simulink model "linealidad"  (R2020b)
settings: Solver=VariableStepAuto  StartTime=0.0  StopTime=5  RelTol=1e-3
settings Model: Creator=carma  LastModifiedBy=carma

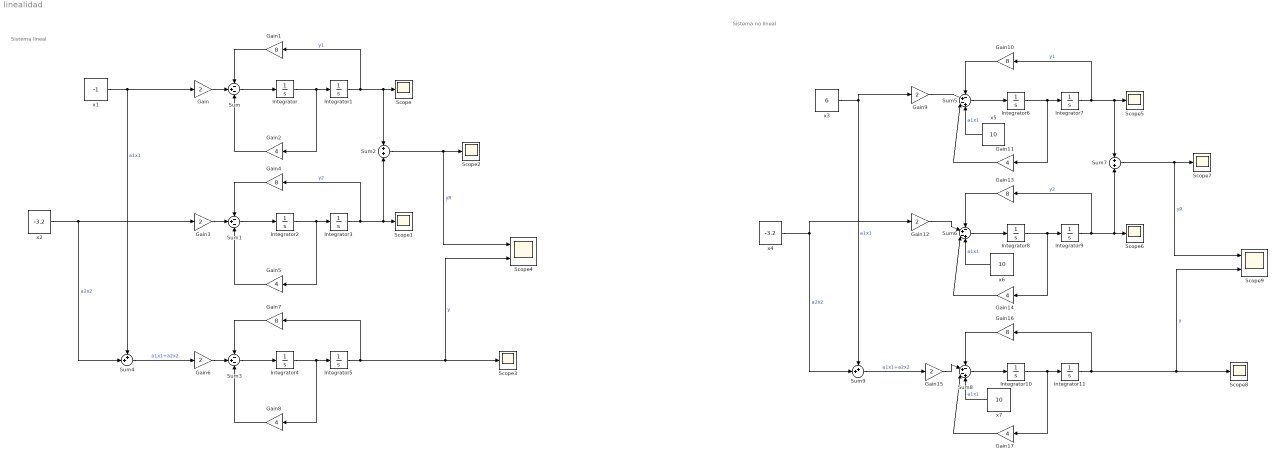
== system linealidad ==
  note: Sistema no lineal
  note: Sistema lineal
  Gain{,3,6,9,12,15} (6 alike) : Gain  Gain=2
  Gain{1,4,7,10,13,16} (6 alike) : Gain  Gain=8
  Gain{2,5,8,11,14,17} (6 alike) : Gain  Gain=4
  Integrator{,1..11} (12 alike) : Integrator
  Scope{,1..3,5..8} (8 alike) : Scope
  Scope4 : Scope  NumInputPorts=2
  Scope9 : Scope  NumInputPorts=2
  Sum : Sum  Inputs=-+-
  Sum1 : Sum  Inputs=-+-
  Sum2 : Sum
  Sum3 : Sum  Inputs=-+-
  Sum4 : Sum  Inputs=++|
  Sum5 : Sum  Inputs=-+-+
  Sum6 : Sum  Inputs=-+-+
  Sum7 : Sum
  Sum8 : Sum  Inputs=-+-+
  Sum9 : Sum  Inputs=++|
  x1 : Constant  Value=-1  VectorParams1D=off  SampleTime=-1
  x2 : Constant  Value=-3.2  VectorParams1D=off  SampleTime=-1
  x3 : Constant  Value=6  VectorParams1D=off  SampleTime=-1
  x4 : Constant  Value=-3.2  VectorParams1D=off  SampleTime=-1
  x5 : Constant  Value=10  VectorParams1D=off  SampleTime=-1
  x6 : Constant  Value=10  VectorParams1D=off  SampleTime=-1
  x7 : Constant  Value=10  VectorParams1D=off  SampleTime=-1
  wires:
  Gain/1 -> Sum/2
  Gain1/1 -> Sum/1
  Gain2/1 -> Sum/3
  Sum/1 -> Integrator/1
  Integrator/1 -> Gain2/1, Integrator1/1
  Integrator1/1 -> Sum2/1, Scope/1, Gain1/1  "y1"
  x1/1 -> Sum4/1, Gain/1  "a1x1"
  Gain3/1 -> Sum1/2
  x2/1 -> Sum4/2, Gain3/1  "a2x2"
  Sum1/1 -> Integrator2/1
  Integrator3/1 -> Sum2/2, Scope1/1, Gain4/1  "y2"
  Gain5/1 -> Sum1/3
  Integrator2/1 -> Gain5/1, Integrator3/1
  Gain4/1 -> Sum1/1
  Sum2/1 -> Scope4/1, Scope2/1  "yR"
  Gain6/1 -> Sum3/2
  Sum4/1 -> Gain6/1  "a1x1+a2x2"
  Sum3/1 -> Integrator4/1
  Integrator5/1 -> Scope4/2, Scope3/1, Gain7/1  "y"
  Gain8/1 -> Sum3/3
  Integrator4/1 -> Gain8/1, Integrator5/1
  Gain7/1 -> Sum3/1
  Sum9/1 -> Gain15/1  "a1x1+a2x2"
  Sum7/1 -> Scope9/1, Scope7/1  "yR"
  Gain13/1 -> Sum6/1
  Sum6/1 -> Integrator8/1
  Gain14/1 -> Sum6/3
  Gain12/1 -> Sum6/2
  x4/1 -> Sum9/2, Gain12/1  "a2x2"
  Gain16/1 -> Sum8/1
  Integrator10/1 -> Gain17/1, Integrator11/1
  Gain17/1 -> Sum8/3
  Gain15/1 -> Sum8/2
  Integrator9/1 -> Sum7/2, Scope6/1, Gain13/1  "y2"
  Sum8/1 -> Integrator10/1
  Gain9/1 -> Sum5/2
  Integrator11/1 -> Scope9/2, Scope8/1, Gain16/1  "y"
  x3/1 -> Sum9/1, Gain9/1  "a1x1"
  Sum5/1 -> Integrator6/1
  Integrator7/1 -> Sum7/1, Scope5/1, Gain10/1  "y1"
  Gain11/1 -> Sum5/3
  Integrator6/1 -> Gain11/1, Integrator7/1
  Gain10/1 -> Sum5/1
  Integrator8/1 -> Gain14/1, Integrator9/1
  x5/1 -> Sum5/4  "a1x1"
  x6/1 -> Sum6/4  "a1x1"
  x7/1 -> Sum8/4  "a1x1"
